simulink model "MBD_W2_P1"  (R2020a)
settings: Solver=VariableStepAuto  StartTime=0.0  StopTime=inf  RelTol=1e-3
settings Model: EnablePacing=on  Creator=Atri Mondal  LastModifiedBy=Atri Mondal

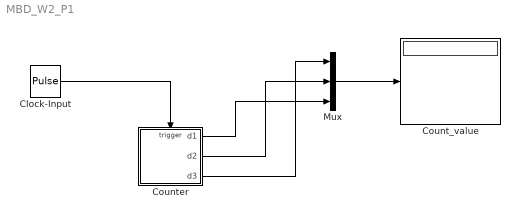
== system MBD_W2_P1 ==
  Clock-Input : DiscretePulseGenerator  PulseType=Time based  Period=1
  Count_value : Display
  Counter : Stateflow chart  TreatAsAtomicUnit=on
  Mux : Mux  Inputs=3
  wires:
  Clock-Input/1 -> Counter/Trigger
  Counter/3(d3) -> Mux/1
  Mux/1 -> Count_value/1
  Counter/1(d1) -> Mux/3
  Counter/2(d2) -> Mux/2

== stateflow chart MBD_W2_P1/Counter ==
  settings: executeAtInitialization=1
  state Mod_5_Counter
    state Digit_1 [parallel]
      settings: executionOrder=1
      state Zero
        en:
        d1=0;
        count=count+1;
      state One
        en:
        d1=1;
        count=count+1;
      (default) -> Mod_5_Counter.Digit_1.Zero
      Mod_5_Counter.Digit_1.Zero -> Mod_5_Counter.Digit_1.One : inputclk
      Mod_5_Counter.Digit_1.One -> Mod_5_Counter.Digit_1.Zero : inputclk /{Digit_2.inc2;}
    state Digit_2 [parallel]
      settings: executionOrder=2
      state Zero
        en:
        d2=0;
      state One
        en:
        d2=1;
      (default) -> Mod_5_Counter.Digit_2.Zero
      Mod_5_Counter.Digit_2.Zero -> Mod_5_Counter.Digit_2.One : inc2
      Mod_5_Counter.Digit_2.One -> Mod_5_Counter.Digit_2.Zero : inc2/{Digit_3.inc3;}
    state Digit_3 [parallel]
      settings: executionOrder=3
      state Zero
        en:
        d3=0;
      state One
        en:
        d3=1;
      (default) -> Mod_5_Counter.Digit_3.Zero
      Mod_5_Counter.Digit_3.Zero -> Mod_5_Counter.Digit_3.One : inc3
  state Init
    en:
    count=0;
  (default) -> Init
  Init -> Mod_5_Counter : [count==0]
  Mod_5_Counter -> Init : [count==5]
  data: d1 output; d2 output; d3 output; count local
  events: inc2 local FUNCTION_CALL_EVENT; inc3 local FUNCTION_CALL_EVENT; inputclk input RISING_EDGE_EVENT
